simulink model "lab1simulink"  (R2020a)
settings: Solver=VariableStepAuto  StartTime=0.0  StopTime=20.0  RelTol=1e-3
settings Model: Creator=Victor  LastModifiedBy=Victor

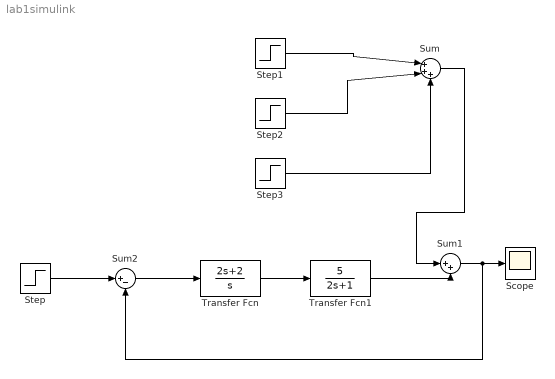
== system lab1simulink ==
  Scope : Scope
  Step : Step  Time=0  After=0  SampleTime=0
  Step1 : Step  Time=3  After=0.2  SampleTime=0
  Step2 : Step  Time=6  After=0.1  SampleTime=0
  Step3 : Step  Time=9  After=0.1  SampleTime=0
  Sum : Sum  Inputs=|+++
  Sum1 : Sum  Inputs=|++
  Sum2 : Sum  Inputs=|+-
  Transfer Fcn : TransferFcn  Numerator=[2 2]  Denominator=[1 0]
  Transfer Fcn1 : TransferFcn  Numerator=[5]  Denominator=[2 1]
  wires:
  Step3/1 -> Sum/3
  Step2/1 -> Sum/2
  Step1/1 -> Sum/1
  Sum/1 -> Sum1/1
  Step/1 -> Sum2/1
  Sum1/1 -> Sum2/2, Scope/1
  Transfer Fcn/1 -> Transfer Fcn1/1
  Transfer Fcn1/1 -> Sum1/2
  Sum2/1 -> Transfer Fcn/1
